simulink model "Coupled_I_eqn"  (R2022a)
settings: Solver=ode45  StartTime=0.0  StopTime=0.5  RelTol=1e-7
settings Model: Creator=Sukruth  LastModifiedBy=Sukruth

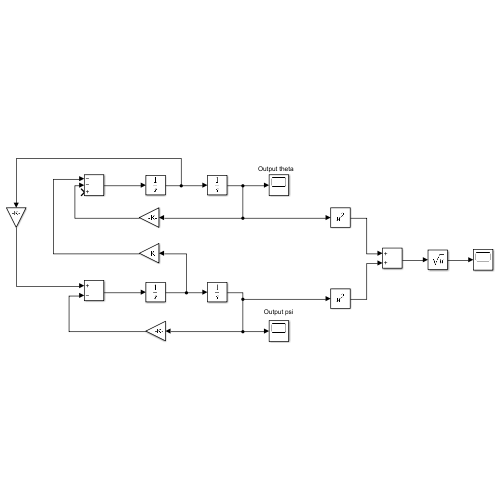
[thumbnail: Simulink's stored preview of the top-level diagram]
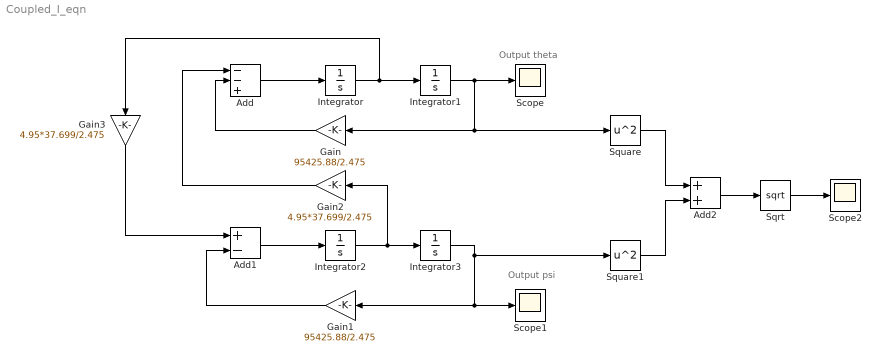
== system Coupled_I_eqn ==
  note: Output psi
  note: Output theta
  Add : Sum  Inputs=--+
  Add1 : Sum  Inputs=+-
  Add2 : Sum
  Gain : Gain  Gain=95425.88/2.475
  Gain1 : Gain  Gain=95425.88/2.475
  Gain2 : Gain  Gain=4.95*37.699/2.475
  Gain3 : Gain  Gain=4.95*37.699/2.475
  Integrator : Integrator
  Integrator1 : Integrator  InitialCondition=pi/10
  Integrator2 : Integrator
  Integrator3 : Integrator  InitialCondition=pi/10
  Scope : Scope
  Scope1 : Scope
  Scope2 : Scope
  Sqrt : Sqrt
  Square : Math  Operator=square
  Square1 : Math  Operator=square
  wires:
  Add/1 -> Integrator/1
  Integrator/1 -> Integrator1/1, Gain3/1
  Add1/1 -> Integrator2/1
  Integrator2/1 -> Gain2/1, Integrator3/1
  Gain/1 -> Add/2
  Gain1/1 -> Add1/2
  Gain2/1 -> Add/1
  Gain3/1 -> Add1/1
  Integrator3/1 -> Square1/1, Gain1/1, Scope1/1
  Add2/1 -> Sqrt/1
  Integrator1/1 -> Scope/1, Gain/1, Square/1
  Sqrt/1 -> Scope2/1
  Square1/1 -> Add2/2
  Square/1 -> Add2/1
